simulink model "three_phase_Gen_SpeedControl_new"  (R2023b)
settings: Solver=FixedStepAuto  StartTime=0.0  StopTime=10  FixedStep=Ts  RelTol=1e-3  EnableMultiTasking=on
undefined symbols (not defined in the file): motor_base_freq, Target, Ts
libraries: svdschedulerlib x2, simulink x2, mcbcontrolslib x2, c280xlib x1
settings Model: ExtModeTrigDuration=8  Creator=ela19kfs  LastModifiedBy=kapis
settings OptimizationCC: DefaultUnderspecifiedDataType=single  EnhancedBackFolding=on  PassReuseOutputArgsAs=Individual arguments  MaxStackSize=1024  OptimizeBlockOrder=speed  DifferentSizesBufferReuse=on  OptimizationCustomize=off  EfficientTunableParamExpr=on
settings DebuggingCC: ParameterPrecisionLossMsg=none  ParameterTunabilityLossMsg=error
settings HardwareCC: ProdBitPerChar=16  ProdBitPerInt=16  ProdBitPerPointer=32  ProdBitPerSizeT=32  ProdBitPerPtrDiffT=32  ProdLargestAtomicInteger=Integer  ProdLargestAtomicFloat=None  ProdWordSize=16  ProdLongLongMode=on  ProdHWDeviceType=Texas Instruments->C2000  HardwareBoardFeatureSet=SoCBlockset
settings ModelReferenceCC: ModelReferenceNumInstancesAllowed=Single
settings SFSimCC: MATLABDynamicMemAlloc=off
settings RTWCC: Description=Embedded Coder  SystemTargetFile=ert.tlc  HardwareBoard=TI Delfino F2837xD  TemplateMakefile=ert_default_tmf  Toolchain=Texas Instruments Code Composer Studio (C2000)  CodeProfilingSaveOptions=MetricsOnly
settings CodeAppCC: ForceParamTrailComments=on  IgnoreCustomStorageClasses=off  OperatorAnnotations=on  SimulinkDataObjDesc=on  SFDataObjDesc=on  InsertBlockDesc=on
settings ERTTargetCC: CodeReplacementLibrary=TI C28x  ExtModeTransport=4  ExtModeStaticAlloc=on  ExtModeAutomaticAllocSize=off  ExtModeStaticAllocSize=10000  ExtModeMexFile=ext_xcp  ExtModeIntrfLevel=Level2 - Open

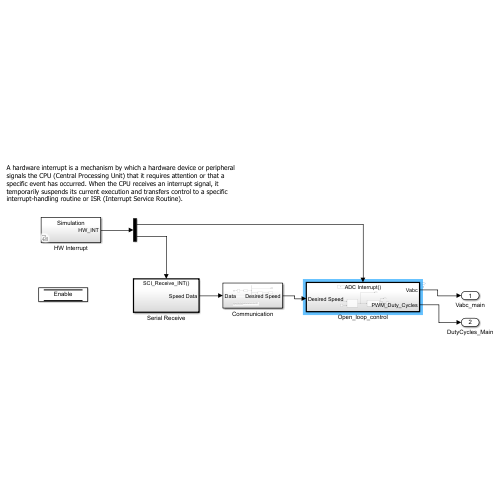
[thumbnail: Simulink's stored preview of the top-level diagram]
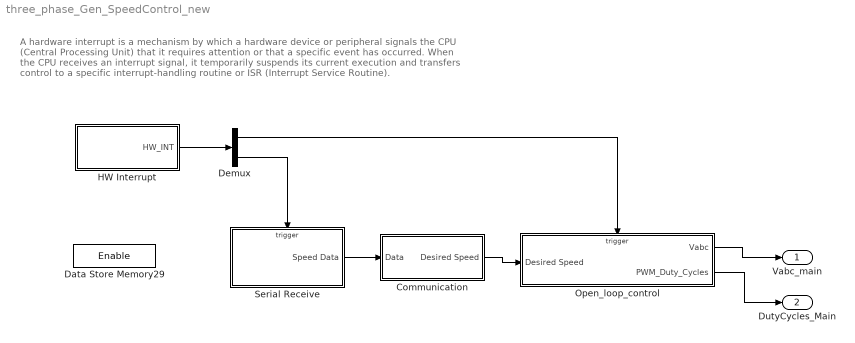
== system three_phase_Gen_SpeedControl_new ==
  note: A hardware interrupt is a mechanism by which a hardware device or peripheral signals the CPU (Central Processing Unit) that it requires attention or that a specific event has occurred. When the CPU receives an interrupt signal, it temporarily suspends its current execution and transfers control to a specific interrupt-handling routine or ISR (Interrupt Service Routine).
  Communication : Subsystem
  Data Store Memory29 : DataStoreMemory  DataStoreName=Enable  ShowAdditionalParam=off  OutDataTypeStr=boolean
  Demux : Demux  Outputs=2
  HW Interrupt : Subsystem  Variant=on  VariantControlMode=sim codegen switching
  Open_loop_control : Subsystem
  Serial Receive : Subsystem  SystemSampleTime=1e-3
      settings: RTWSystemCode=Nonreusable function
  Vabc_main : Outport
  DutyCycles_Main : Outport  Port=2
  wires:
  HW Interrupt/1(HW_INT) -> Demux/1
  Demux/2 -> Serial Receive/Trigger
  Demux/1 -> Open_loop_control/Trigger
  Serial Receive/1(Speed Data) -> Communication/1(Data)
  Communication/1(Desired Speed) -> Open_loop_control/1(Desired Speed)
  Open_loop_control/1(Vabc) -> Vabc_main/1
  Open_loop_control/2(PWM_Duty_Cycles) -> DutyCycles_Main/1

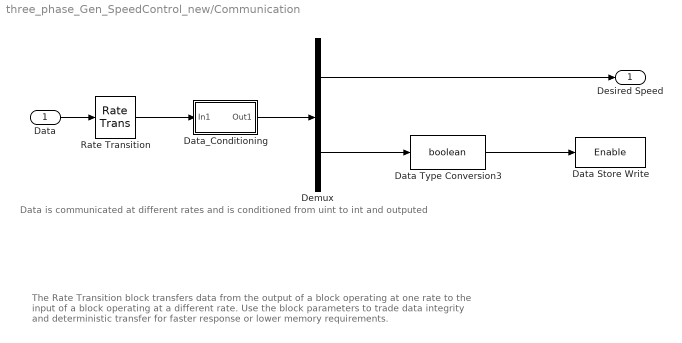
== system three_phase_Gen_SpeedControl_new/Communication ==
  note: The Rate Transition block transfers data from the output of a block operating at one rate to the input of a block operating at a different rate. Use the block parameters to trade data integrity and deterministic transfer for faster response or lower memory requirements.
  note: Data is communicated at different rates and is conditioned from uint to int and outputed
  Data : Inport
  Data Store Write : DataStoreWrite  DataStoreName=Enable  IndexOptions=Index vector (dialog)  Indices=1  OutputSizes=1
  Data Type Conversion3 : DataTypeConversion  OutDataTypeStr=boolean  RndMeth=Simplest  SaturateOnIntegerOverflow=off
  Data_Conditioning : Subsystem
  Demux : Demux  Outputs=2
  Rate Transition : RateTransition  Deterministic=off  InitialCondition=[1228 0]  OutPortSampleTime=Ts
  Desired Speed : Outport  VectorParamsAs1DForOutWhenUnconnected=off
  wires:
  Rate Transition/1 -> Data_Conditioning/1(In1)
  Data_Conditioning/1(Out1) -> Demux/1
  Demux/1 -> Desired Speed/1
  Data Type Conversion3/1 -> Data Store Write/1
  Demux/2 -> Data Type Conversion3/1
  Data/1 -> Rate Transition/1

== system three_phase_Gen_SpeedControl_new/HW Interrupt ==
  Code generation : Subsystem  VariantControl=(codegen)
  Simulation : Subsystem  VariantControl=(sim)
  HW_INT : Outport  OutputFunctionCall=on

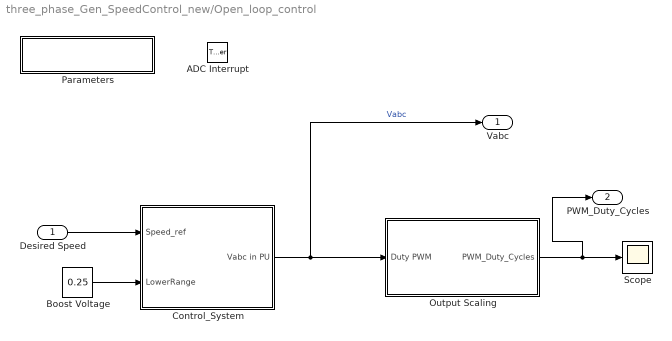
== system three_phase_Gen_SpeedControl_new/Open_loop_control ==
  Desired Speed : Inport
  ADC Interrupt : TriggerPort  TriggerType=function-call  VariantControl=Variant
  Boost Voltage : Constant  Value=0.25  OutDataTypeStr=single
  Control_System : Subsystem
  Output Scaling : Subsystem
  Parameters : Subsystem
  Scope : Scope
  Vabc : Outport
  PWM_Duty_Cycles : Outport  Port=2
  wires:
  Desired Speed/1 -> Control_System/1(Speed_ref)
  Control_System/1(Vabc in PU) -> Output Scaling/1(Duty PWM), Vabc/1  "Vabc"
  Boost Voltage/1 -> Control_System/2(LowerRange)
  Output Scaling/1(PWM_Duty_Cycles) -> PWM_Duty_Cycles/1, Scope/1

== system three_phase_Gen_SpeedControl_new/Serial Receive ==
  note: Received Data from the MCU SCI pin
  SCI_Receive_INT : TriggerPort  TriggerType=function-call  VariantControl=Variant
  SCI_Rx : Subsystem  Variant=on  VariantControlMode=sim codegen switching
  Speed Data : Outport  VectorParamsAs1DForOutWhenUnconnected=off
  wires:
  SCI_Rx/1(Output) -> Speed Data/1

== system three_phase_Gen_SpeedControl_new/Communication/Data_Conditioning ==
  In1 : Inport
  Data Type Conversion2 : DataTypeConversion  OutDataTypeStr=int16  ConvertRealWorld=Stored Integer (SI)  RndMeth=Simplest  SaturateOnIntegerOverflow=off
  Out1 : Outport  VectorParamsAs1DForOutWhenUnconnected=off
  wires:
  Data Type Conversion2/1 -> Out1/1
  In1/1 -> Data Type Conversion2/1

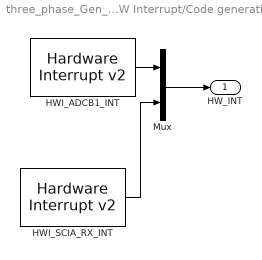
== system three_phase_Gen_SpeedControl_new/HW Interrupt/Code generation ==
  HWI_ADCB1_INT : svdschedulerlib/Hardware Interrupt v2  ISRGroup=ADC - Analog to Digital Converter  ISRName=ADCA1_INT  ISRNumber=32  NumEventsToServe=1  EventsList={'on','EOC event','1';'off','Overflow event','2';'off','Custom event','3'}  SelectedEvents={'event1'}  TaskPriority=30  DisablePreemption=on  ClearInterruptFlagsAtEndOfEvent=on  InterruptDefinitionFile=$(TARGET_ROOT)/registry/interrupts/F2837xS_interrupts.xml  HardwareBoard=F2837x  EnableSimPort=off
      settings: LibrarySourceBlock=c2000lib/Scheduling/Hardware Interrupt
  HWI_SCIA_RX_INT : svdschedulerlib/Hardware Interrupt v2  ISRGroup=ADC - Analog to Digital Converter  ISRName=ADCA1_INT  ISRNumber=32  NumEventsToServe=1  EventsList={'on','EOC event','1';'off','Overflow event','2';'off','Custom event','3'}  SelectedEvents={'event1'}  TaskPriority=50  DisablePreemption=off  ClearInterruptFlagsAtEndOfEvent=on  InterruptDefinitionFile=$(TARGET_ROOT)/registry/interrupts/F2837xS_interrupts.xml  HardwareBoard=F2837x  EnableSimPort=off
      settings: LibrarySourceBlock=c2000lib/Scheduling/Hardware Interrupt
  Mux : Mux  Inputs=2
  HW_INT : Outport
  wires:
  HWI_ADCB1_INT/1 -> Mux/1
  Mux/1 -> HW_INT/1
  HWI_SCIA_RX_INT/1 -> Mux/2

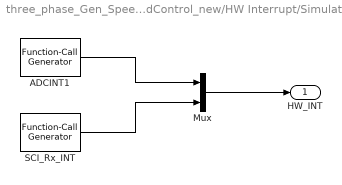
== system three_phase_Gen_SpeedControl_new/HW Interrupt/Simulation ==
  ADCINT1 : simulink/Ports & Subsystems/Function-Call Generator  sample_time=Ts  numberOfIterations=1  DisallowWideOutput=off
  Mux : Mux  Inputs=2
  SCI_Rx_INT : simulink/Ports & Subsystems/Function-Call Generator  sample_time=0.1  numberOfIterations=1  DisallowWideOutput=off
  HW_INT : Outport
  wires:
  SCI_Rx_INT/1 -> Mux/2
  ADCINT1/1 -> Mux/1
  Mux/1 -> HW_INT/1

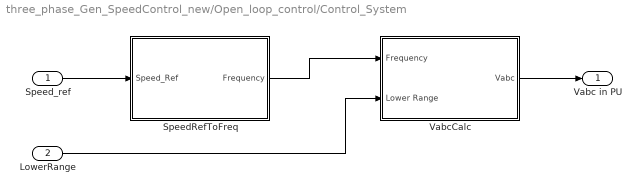
== system three_phase_Gen_SpeedControl_new/Open_loop_control/Control_System ==
  Speed_ref : Inport
  LowerRange : Inport  Port=2
  SpeedRefToFreq : Subsystem
  VabcCalc : Subsystem
  Vabc in PU : Outport  VectorParamsAs1DForOutWhenUnconnected=off
  wires:
  Speed_ref/1 -> SpeedRefToFreq/1(Speed_Ref)
  SpeedRefToFreq/1(Frequency) -> VabcCalc/1(Frequency)
  VabcCalc/1(Vabc) -> Vabc in PU/1
  LowerRange/1 -> VabcCalc/2(Lower Range)

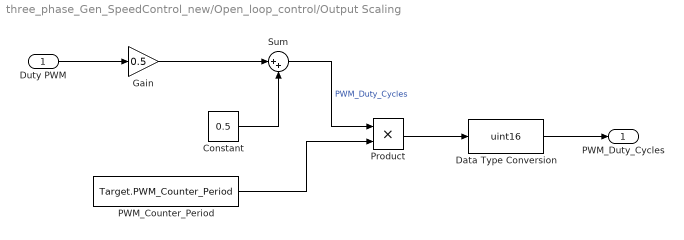
== system three_phase_Gen_SpeedControl_new/Open_loop_control/Output Scaling ==
  Duty PWM : Inport
  Constant : Constant  Value=0.5  OutDataTypeStr=single
  Data Type Conversion : DataTypeConversion  OutDataTypeStr=uint16  SaturateOnIntegerOverflow=off  RndMeth=Floor
  Gain : Gain  Gain=0.5  OutDataTypeStr=Inherit: Same as input
  PWM_Counter_Period : Constant  Value=Target.PWM_Counter_Period  OutDataTypeStr=dataType  SampleTime=-1
  Product : Product
  Sum : Sum  Inputs=|++  OutDataTypeStr=single
  PWM_Duty_Cycles : Outport
  wires:
  Constant/1 -> Sum/2
  Duty PWM/1 -> Gain/1
  Gain/1 -> Sum/1
  Sum/1 -> Product/1  "PWM_Duty_Cycles"
  PWM_Counter_Period/1 -> Product/2
  Data Type Conversion/1 -> PWM_Duty_Cycles/1
  Product/1 -> Data Type Conversion/1

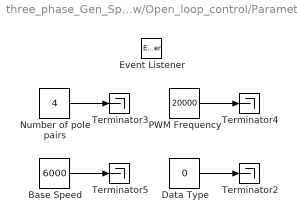
== system three_phase_Gen_SpeedControl_new/Open_loop_control/Parameters ==
  Base Speed : Constant  Value=6000
  Data Type : Constant  Value=0
  Event Listener : EventListener  DisableCoverage=on  EventName=reset
  Number of pole pairs : Constant  Value=4
  PWM Frequency : Constant  Value=20000
  Terminator{2..5} (4 alike) : Terminator
  wires:
  Data Type/1 -> Terminator2/1
  Number of pole pairs/1 -> Terminator3/1
  PWM Frequency/1 -> Terminator4/1
  Base Speed/1 -> Terminator5/1

== system three_phase_Gen_SpeedControl_new/Serial Receive/SCI_Rx ==
  Codegen : Subsystem  VariantControl=(codegen)
  Sim : Subsystem  VariantControl=(sim)
  Output : Outport

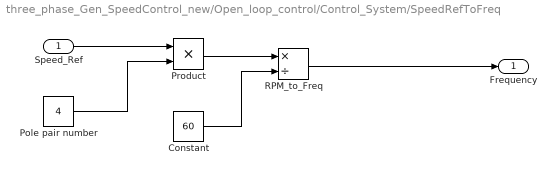
== system three_phase_Gen_SpeedControl_new/Open_loop_control/Control_System/SpeedRefToFreq ==
  Speed_Ref : Inport
  Constant : Constant  Value=60  OutDataTypeStr=single
  Pole pair number : Constant  Value=4  OutDataTypeStr=single
  Product : Product
  RPM_to_Freq : Product  Inputs=*/  OutDataTypeStr=single
  Frequency : Outport
  wires:
  Speed_Ref/1 -> Product/1
  Pole pair number/1 -> Product/2
  Product/1 -> RPM_to_Freq/1
  Constant/1 -> RPM_to_Freq/2
  RPM_to_Freq/1 -> Frequency/1

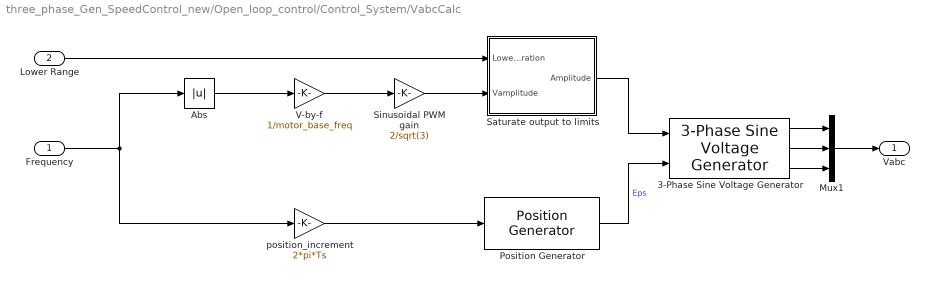
== system three_phase_Gen_SpeedControl_new/Open_loop_control/Control_System/VabcCalc ==
  Frequency : Inport
  Lower Range : Inport  Port=2
  3-Phase Sine Voltage Generator : mcbcontrolslib/3-Phase Sine Voltage Generator  AngleInput=Radians  N_points=1024
  Abs : Abs  RndMeth=Simplest  SaturateOnIntegerOverflow=off
  Mux1 : Mux  Inputs=3
  Position Generator : mcbcontrolslib/Position Generator  AngleOutput=Radians  ExternalReset=none  Offset=0
  Saturate output to limits : Subsystem
  Sinusoidal PWM gain : Gain  Gain=2/sqrt(3)  RndMeth=Simplest  OutDataTypeStr=Inherit: Same as input
  V-by-f : Gain  Gain=1/motor_base_freq  RndMeth=Simplest  OutDataTypeStr=Inherit: Same as input
  position_increment : Gain  Gain=2*pi*Ts  RndMeth=Simplest  OutDataTypeStr=Inherit: Same as input
  Vabc : Outport
  wires:
  Frequency/1 -> Abs/1, position_increment/1
  position_increment/1 -> Position Generator/1
  3-Phase Sine Voltage Generator/3 -> Mux1/3
  3-Phase Sine Voltage Generator/2 -> Mux1/2
  V-by-f/1 -> Sinusoidal PWM gain/1
  3-Phase Sine Voltage Generator/1 -> Mux1/1
  Sinusoidal PWM gain/1 -> Saturate output to limits/2(Vamplitude)
  Mux1/1 -> Vabc/1
  Lower Range/1 -> Saturate output to limits/1(Lower Saturation)
  Saturate output to limits/1(Amplitude) -> 3-Phase Sine Voltage Generator/1
  Position Generator/1 -> 3-Phase Sine Voltage Generator/2  "Eps"
  Abs/1 -> V-by-f/1

== system three_phase_Gen_SpeedControl_new/Serial Receive/SCI_Rx/Codegen ==
  SCI Receive : c280xlib/SCI Receive  sciModule=A  dataHead=''  headerCheckMaxCount=16  dataTail=''  dataType=uint16  dataLenOptions=Length via dialog  dataDim=2  maxDataLength=1  initValue=0  errOption=Output the last received value  errValue=0  sampleTime=-1  blockingMode=on  timeOut=0.00875  outputStatus=off
  Output : Outport
  wires:
  SCI Receive/1 -> Output/1

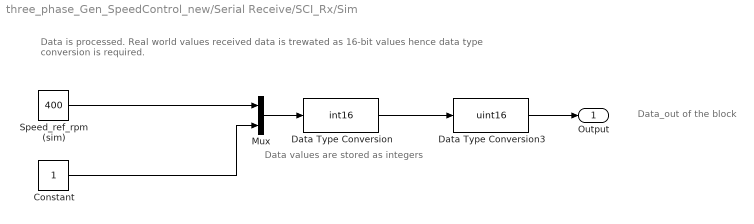
== system three_phase_Gen_SpeedControl_new/Serial Receive/SCI_Rx/Sim ==
  note: Data is processed. Real world values received data is trewated as 16-bit values hence data type conversion is required.
  note: Data values are stored as integers
  note: Data_out of the block
  Constant : Constant  OutDataTypeStr=single
  Data Type Conversion : DataTypeConversion  OutDataTypeStr=int16  SaturateOnIntegerOverflow=off  RndMeth=Floor
  Data Type Conversion3 : DataTypeConversion  OutDataTypeStr=uint16  ConvertRealWorld=Stored Integer (SI)  RndMeth=Simplest  SaturateOnIntegerOverflow=off
  Mux : Mux  Inputs=2
  Speed_ref_rpm (sim) : Constant  Value=400  OutDataTypeStr=single  SampleTime=-1
  Output : Outport
  wires:
  Data Type Conversion3/1 -> Output/1
  Mux/1 -> Data Type Conversion/1
  Constant/1 -> Mux/2
  Speed_ref_rpm (sim)/1 -> Mux/1
  Data Type Conversion/1 -> Data Type Conversion3/1

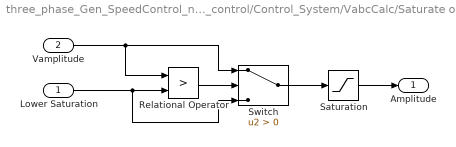
== system three_phase_Gen_SpeedControl_new/Open_loop_control/Control_System/VabcCalc/Saturate output to limits ==
  Lower Saturation : Inport
  Vamplitude : Inport  Port=2
  Relational Operator : RelationalOperator  Operator=>  OutDataTypeStr=boolean  RndMeth=Simplest  InputSameDT=off
  Saturation : Saturate  UpperLimit=0.95  LowerLimit=0  RndMeth=Simplest
  Switch : Switch  Criteria=u2 > Threshold  SaturateOnIntegerOverflow=off  InputSameDT=off
  Amplitude : Outport
  wires:
  Saturation/1 -> Amplitude/1
  Switch/1 -> Saturation/1
  Relational Operator/1 -> Switch/2
  Lower Saturation/1 -> Switch/3, Relational Operator/2
  Vamplitude/1 -> Switch/1, Relational Operator/1
